simulink model "host_programa"  (R2013b)
settings: Solver=FixedStepDiscrete  StartTime=0.00000  StopTime=inf  FixedStep=0.001  MaxStep=0.001  RelTol=1e-3
undefined symbols (not defined in the file): get, hot
libraries: dsparch4 x6, dspsigops x3, dspsnks4 x1
settings Model: MAModelExclusionFile=C:\TFG\Matlab_Files\host_programa_exclusions.xml  Creator=Sr Antonio  LastModifiedBy=gonza
settings DataIOCC: LimitDataPoints=off  SaveFormat=StructureWithTime  InspectSignalLogs=on
settings OptimizationCC: ExpressionDepthLimit=2147483647
settings DebuggingCC: FcnCallInpInsideContextMsg=EnableAllAsWarning  StateNameClashWarn=warning
settings GRTTargetCC: CombineOutputUpdateFcns=off  GRTInterface=on

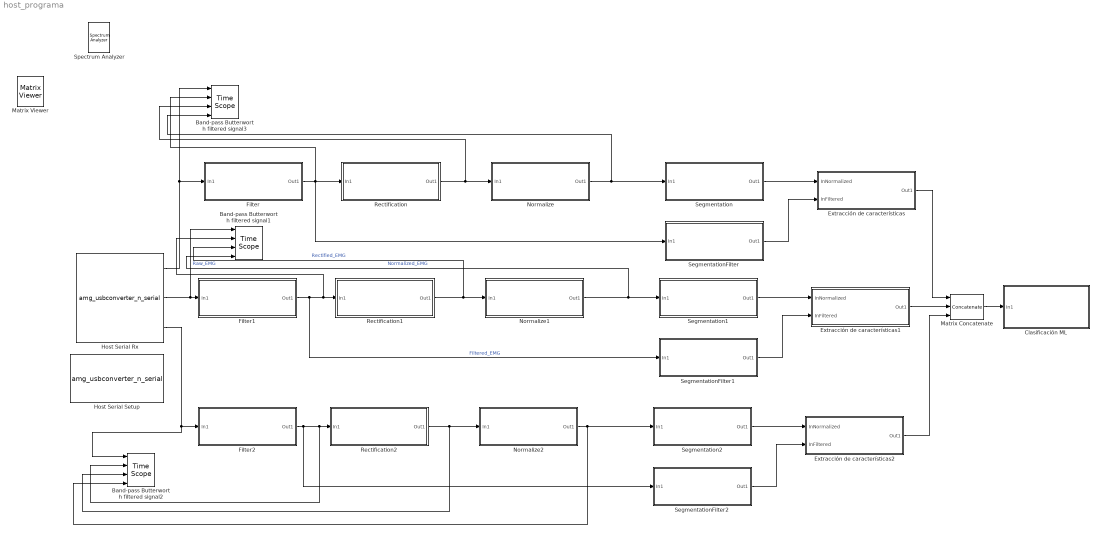
== system host_programa ==
  Band-pass Butterworth filtered signal1 : TimeScope  NumInputPorts=4  DefaultConfigurationName=spbscopes.TimeScopeBlockCfg
      settings: CopyFcn=scopeextensions.ScopeBlock.onCoreBlockCopy(gcbh);  DeleteFcn=scopeextensions.ScopeBlock.callback(gcbh, 'onBlockDelete');  PreSaveFcn=scopeextensions.ScopeBlock.callback(gcbh, 'onModelSave');  NameChangeFcn=scopeextensions.ScopeBlock.callback(gcbh, 'onBlockRename');  DestroyFcn=scopeextensions.ScopeBlock.onBlockDestroy(gcbh)  CloseFcn=scopeextensions.ScopeBlock.callback(gcbh, 'onBlockClose');  PreDeleteFcn=scopeextensions.ScopeBlock.callback(gcbh, 'onBlockPreDelete');
  Band-pass Butterworth filtered signal2 : TimeScope  NumInputPorts=4  DefaultConfigurationName=spbscopes.TimeScopeBlockCfg
      settings: CopyFcn=scopeextensions.ScopeBlock.onCoreBlockCopy(gcbh);  DeleteFcn=scopeextensions.ScopeBlock.callback(gcbh, 'onBlockDelete');  PreSaveFcn=scopeextensions.ScopeBlock.callback(gcbh, 'onModelSave');  NameChangeFcn=scopeextensions.ScopeBlock.callback(gcbh, 'onBlockRename');  DestroyFcn=scopeextensions.ScopeBlock.onBlockDestroy(gcbh)  CloseFcn=scopeextensions.ScopeBlock.callback(gcbh, 'onBlockClose');  PreDeleteFcn=scopeextensions.ScopeBlock.callback(gcbh, 'onBlockPreDelete');
  Band-pass Butterworth filtered signal3 : TimeScope  NumInputPorts=4  DefaultConfigurationName=spbscopes.TimeScopeBlockCfg
      settings: CopyFcn=scopeextensions.ScopeBlock.onCoreBlockCopy(gcbh);  DeleteFcn=scopeextensions.ScopeBlock.callback(gcbh, 'onBlockDelete');  PreSaveFcn=scopeextensions.ScopeBlock.callback(gcbh, 'onModelSave');  NameChangeFcn=scopeextensions.ScopeBlock.callback(gcbh, 'onBlockRename');  DestroyFcn=scopeextensions.ScopeBlock.onBlockDestroy(gcbh)  CloseFcn=scopeextensions.ScopeBlock.callback(gcbh, 'onBlockClose');  PreDeleteFcn=scopeextensions.ScopeBlock.callback(gcbh, 'onBlockPreDelete');
  Clasificación ML : Subsystem
  Extracción de características : Subsystem
  Extracción de características1 : Subsystem
  Extracción de características2 : Subsystem
  Filter : Subsystem
  Filter1 : Subsystem
  Filter2 : Subsystem
  Host Serial Rx : S-Function  Priority=1  FunctionName=amg_usbconverter_n_serial  Parameters=configuration,port,transfer,baudrate,stopbit,inputtype,outputtype,binheaderarray,binterminatorarray,asciiheader,asciiterminator,bindatalength,packetmode,timeout,sampletime,sampletimestr,blockid  EnableBusSupport=off  mask(amg_usbconverter_n_serial){configuration=Rx, port=COM3, baudrate=115200, databits=8, parity=None, stopbit=1, flowcontrol=None, advanceoptions=off, rxbuffersize=2048, txbuffersize=2048, transfer=Blocking, timeout=2, packetmode=Binary, binheader='0E 0E', binterminator='0A 0A', porttype_double=0, porttype_single=3, porttype_int8=0, porttype_uint8=0, porttype_int16=0, porttype_uint16=0, porttype_int32=0, porttype_uint32=0, asciiformat='%d,%f', rx_asciiterminator=LF (0x0A - "\n"), tx_asciiterminator=LF (0x0A - "\n"), inputtype=[0], outputtype=[3  1 1 1], binheaderarray=[2 14  14], binterminatorarray=[2 10  10], bindatalength=12, asciiheader=['%d,%f' uint8(10)], asciiterminator=[1 10], sampletime=0.001, sampletimestr=, blockid=HostSerialRx}
      mask prompts: baudrate "Baud rate (bps)"; databits "Data bits"; stopbit "Stop bit"; flowcontrol "Hardware flow control"; advanceoptions "Advance options"; rxbuffersize "Rx buffer size (bytes)"; txbuffersize "Tx buffer size (bytes)"; timeout "Wait time-out (Seconds)"; packetmode "Packet mode"; binheader "Binary header (example: '7E 7E')"; binterminator "Binary terminator (example: '03 03')"; porttype_double "Number of data port, type DOUBLE"; porttype_single "Number of data port, type SINGLE"; porttype_int8 "Number of data port, type INT8"; porttype_uint8 "Number of data port, type UINT8"; porttype_int16 "Number of data port, type INT16"; porttype_uint16 "Number of data port, type UINT16"; porttype_int32 "Number of data port, type INT32"; porttype_uint32 "Number of data port, type UINT32"; asciiformat "Ascii format"; rx_asciiterminator "End of packet"; tx_asciiterminator "End of packet"; inputtype "Input data type"; outputtype "Output data type"; binheaderarray "Binary header"; binterminatorarray "Binary terminator"; bindatalength "Binary data length"; asciiheader "Ascii header (printf format)"; asciiterminator "Ascii terminator"; sampletime "Sample time (sec)"; sampletimestr "Compiled sample time (sec) in string"
      mask init:
      | amg_usbconverter_n_serial_callback('init');
      mask Help: web(fullfile(waijungdocroot,'amg_usbconverter_n_uart.htm'), '-browser')
      mask TypeOptions configuration: Setup | Tx | Rx
      mask Callback configuration: amg_usbconverter_n_serial_callback('configuration');
      mask TypeOptions port: COM3
      mask Callback port: amg_usbconverter_n_serial_callback('port');
      mask Callback baudrate: amg_usbconverter_n_serial_callback('baudrate');
      mask TypeOptions databits: 8
      mask TypeOptions parity: None
      mask TypeOptions stopbit: 1 | 1.5 | 2
      mask TypeOptions flowcontrol: None | RTS | CTS | RTS/CTS
      mask Callback flowcontrol: amg_usbconverter_n_serial_callback('flowcontrol');
      mask Callback advanceoptions: amg_usbconverter_n_serial_callback('advanceoptions');
      mask TypeOptions rxbuffersize: 16 | 32 | 64 | 128 | 256 | 512 | 1024 | 2048
      mask TypeOptions txbuffersize: 16 | 32 | 64 | 128 | 256 | 512 | 1024 | 2048
      mask TypeOptions transfer: Blocking | Non-Blocking
      mask Callback transfer: amg_usbconverter_n_serial_callback('transfer');
      mask TypeOptions packetmode: Ascii | Binary
      mask Callback packetmode: amg_usbconverter_n_serial_callback('packetmode');
      mask Callback binheader: amg_usbconverter_n_serial_callback('binheader');
      mask Callback binterminator: amg_usbconverter_n_serial_callback('binterminator');
      mask Callback porttype_double: amg_usbconverter_n_serial_callback('porttype');
      mask Callback porttype_single: amg_usbconverter_n_serial_callback('porttype');
      mask Callback porttype_int8: amg_usbconverter_n_serial_callback('porttype');
      mask Callback porttype_uint8: amg_usbconverter_n_serial_callback('porttype');
      mask Callback porttype_int16: amg_usbconverter_n_serial_callback('porttype');
      mask Callback porttype_uint16: amg_usbconverter_n_serial_callback('porttype');
      mask Callback porttype_int32: amg_usbconverter_n_serial_callback('porttype');
      mask Callback porttype_uint32: amg_usbconverter_n_serial_callback('porttype');
      mask Callback asciiformat: amg_usbconverter_n_serial_callback('asciiformat');
      mask TypeOptions rx_asciiterminator: CR (0x0D - "\r") | LF (0x0A - "\n") | CRLF (0x0D 0x0A - "\r\n")
      mask Callback rx_asciiterminator: amg_usbconverter_n_serial_callback('rx_asciiterminator');
      mask TypeOptions tx_asciiterminator: CR (0x0D - "\r") | LF (0x0A - "\n") | CRLF (0x0D 0x0A - "\r\n") | None
      mask Callback tx_asciiterminator: amg_usbconverter_n_serial_callback('tx_asciiterminator');
      mask Callback sampletime: amg_usbconverter_n_serial_callback('sampletime');
      mask Callback sampletimestr: amg_usbconverter_n_serial_callback('sampletimestr');
      mask Callback blockid: amg_usbconverter_n_serial_callback('blockid');
      mask Display: text(0.05, 0.5, 'Obsolete !!!\nPort: COM3\nPacket: Binary\nTransfer: Blocking\nTs (sec): 0','ver','middle','hor','left');port_label('output', 1,'single');port_label('output', 2,'single');port_label('output', 3,'single');
  Host Serial Setup : S-Function  Priority=1  FunctionName=amg_usbconverter_n_serial  Parameters=configuration,port,transfer,baudrate,stopbit,inputtype,outputtype,binheaderarray,binterminatorarray,asciiheader,asciiterminator,bindatalength,packetmode,timeout,sampletime,sampletimestr,blockid  EnableBusSupport=off  mask(amg_usbconverter_n_serial){configuration=Setup, port=COM3, baudrate=10000000, databits=8, parity=None, stopbit=1, flowcontrol=None, advanceoptions=off, rxbuffersize=2048, txbuffersize=2048, transfer=Blocking, timeout=5, packetmode=Binary, binheader='7E 7E', binterminator='03 03', porttype_double=1, porttype_single=0, porttype_int8=1, porttype_uint8=0, porttype_int16=0, porttype_uint16=0, porttype_int32=0, porttype_uint32=0, asciiformat='%d,%f', rx_asciiterminator=CRLF (0x0D 0x0A - "\r\n"), tx_asciiterminator=CR (0x0D - "\r"), inputtype=[0], outputtype=[0], binheaderarray=[2 126  126], binterminatorarray=[2 3  3], bindatalength=0, asciiheader='', asciiterminator=[0], sampletime=inf, sampletimestr=, blockid=HostSerialSetup}
      mask prompts: baudrate "Baud rate (bps)"; databits "Data bits"; stopbit "Stop bit"; flowcontrol "Hardware flow control"; advanceoptions "Advance options"; rxbuffersize "Rx buffer size (bytes)"; txbuffersize "Tx buffer size (bytes)"; timeout "Wait time-out (Seconds)"; packetmode "Packet mode"; binheader "Binary header (example: '7E 7E')"; binterminator "Binary terminator (example: '03 03')"; porttype_double "Number of data port, type DOUBLE"; porttype_single "Number of data port, type SINGLE"; porttype_int8 "Number of data port, type INT8"; porttype_uint8 "Number of data port, type UINT8"; porttype_int16 "Number of data port, type INT16"; porttype_uint16 "Number of data port, type UINT16"; porttype_int32 "Number of data port, type INT32"; porttype_uint32 "Number of data port, type UINT32"; asciiformat "Ascii format"; rx_asciiterminator "End of packet"; tx_asciiterminator "End of packet"; inputtype "Input data type"; outputtype "Output data type"; binheaderarray "Binary header"; binterminatorarray "Binary terminator"; bindatalength "Binary data length"; asciiheader "Ascii header (printf format)"; asciiterminator "Ascii terminator"; sampletime "Sample time (sec)"; sampletimestr "Compiled sample time (sec) in string"
      mask init:
      | amg_usbconverter_n_serial_callback('init');
      mask Help: web(fullfile(waijungdocroot,'amg_usbconverter_n_uart.htm'), '-browser')
      mask TypeOptions configuration: Setup | Tx | Rx
      mask Callback configuration: amg_usbconverter_n_serial_callback('configuration');
      mask TypeOptions port: COM3
      mask Callback port: amg_usbconverter_n_serial_callback('port');
      mask Callback baudrate: amg_usbconverter_n_serial_callback('baudrate');
      mask TypeOptions databits: 8
      mask TypeOptions parity: None
      mask TypeOptions stopbit: 1 | 1.5 | 2
      mask TypeOptions flowcontrol: None | RTS | CTS | RTS/CTS
      mask Callback flowcontrol: amg_usbconverter_n_serial_callback('flowcontrol');
      mask Callback advanceoptions: amg_usbconverter_n_serial_callback('advanceoptions');
      mask TypeOptions rxbuffersize: 16 | 32 | 64 | 128 | 256 | 512 | 1024 | 2048
      mask TypeOptions txbuffersize: 16 | 32 | 64 | 128 | 256 | 512 | 1024 | 2048
      mask TypeOptions transfer: Blocking | Non-Blocking
      mask Callback transfer: amg_usbconverter_n_serial_callback('transfer');
      mask TypeOptions packetmode: Ascii | Binary
      mask Callback packetmode: amg_usbconverter_n_serial_callback('packetmode');
      mask Callback binheader: amg_usbconverter_n_serial_callback('binheader');
      mask Callback binterminator: amg_usbconverter_n_serial_callback('binterminator');
      mask Callback porttype_double: amg_usbconverter_n_serial_callback('porttype');
      mask Callback porttype_single: amg_usbconverter_n_serial_callback('porttype');
      mask Callback porttype_int8: amg_usbconverter_n_serial_callback('porttype');
      mask Callback porttype_uint8: amg_usbconverter_n_serial_callback('porttype');
      mask Callback porttype_int16: amg_usbconverter_n_serial_callback('porttype');
      mask Callback porttype_uint16: amg_usbconverter_n_serial_callback('porttype');
      mask Callback porttype_int32: amg_usbconverter_n_serial_callback('porttype');
      mask Callback porttype_uint32: amg_usbconverter_n_serial_callback('porttype');
      mask Callback asciiformat: amg_usbconverter_n_serial_callback('asciiformat');
      mask TypeOptions rx_asciiterminator: CR (0x0D - "\r") | LF (0x0A - "\n") | CRLF (0x0D 0x0A - "\r\n")
      mask Callback rx_asciiterminator: amg_usbconverter_n_serial_callback('rx_asciiterminator');
      mask TypeOptions tx_asciiterminator: CR (0x0D - "\r") | LF (0x0A - "\n") | CRLF (0x0D 0x0A - "\r\n") | None
      mask Callback tx_asciiterminator: amg_usbconverter_n_serial_callback('tx_asciiterminator');
      mask Callback sampletime: amg_usbconverter_n_serial_callback('sampletime');
      mask Callback sampletimestr: amg_usbconverter_n_serial_callback('sampletimestr');
      mask Callback blockid: amg_usbconverter_n_serial_callback('blockid');
      mask Display: text(0.5, 0.5, 'Port: COM3\nBaud (Bps): 10000000\nFrame: 8-None-1','ver','middle','hor','center');
  Matrix Concatenate : Concatenate  NumInputs=3  ConcatenateDimension=2
  Normalize : Subsystem
  Normalize1 : Subsystem
  Normalize2 : Subsystem
  Rectification : Subsystem
  Rectification1 : Subsystem
  Rectification2 : Subsystem
  Segmentation : Subsystem
  Segmentation1 : Subsystem
  Segmentation2 : Subsystem
  SegmentationFilter : Subsystem
  SegmentationFilter1 : Subsystem
  SegmentationFilter2 : Subsystem
  Matrix Viewer : dspsnks4/Matrix Viewer  IOType=viewer  ImageParams=off  CMapStr=hot(256)  AxisColorbar=on  AxisParams=off  AxisOrigin=Upper left corner  XLabel=X-axis  YLabel=Y-axis  ZLabel=Z-axis  FigPos=get(0,'defaultfigureposition')  AxisZoom=off
      settings: YMin=-1.0  YMax=1.0
  Spectrum Analyzer : SpectrumAnalyzer  IOType=viewer
      settings: CopyFcn=scopeextensions.ScopeBlock.onCoreBlockCopy(gcbh);  DeleteFcn=scopeextensions.ScopeBlock.callback(gcbh, 'onBlockDelete');  PreSaveFcn=scopeextensions.ScopeBlock.callback(gcbh, 'onModelSave');  NameChangeFcn=scopeextensions.ScopeBlock.callback(gcbh, 'onBlockRename');  DestroyFcn=scopeextensions.ScopeBlock.onBlockDestroy(gcbh)  CloseFcn=scopeextensions.ScopeBlock.callback(gcbh, 'onBlockClose');  PreDeleteFcn=scopeextensions.ScopeBlock.callback(gcbh, 'onBlockPreDelete');
  wires:
  Host Serial Rx/2 -> Band-pass Butterworth filtered signal1/1, Filter1/1(In1)  "Raw_EMG"
  Filter/1(Out1) -> SegmentationFilter/1(In1), Band-pass Butterworth filtered signal3/2, Rectification/1(In1)
  Filter1/1(Out1) -> SegmentationFilter1/1(In1), Band-pass Butterworth filtered signal1/2, Rectification1/1(In1)  "Filtered_EMG"
  Filter2/1(Out1) -> Band-pass Butterworth filtered signal2/2, Rectification2/1(In1), SegmentationFilter2/1(In1)
  Segmentation/1(Out1) -> Extracción de características/1(InNormalized)
  SegmentationFilter/1(Out1) -> Extracción de características/2(InFiltered)
  Rectification/1(Out1) -> Band-pass Butterworth filtered signal3/3, Normalize/1(In1)
  Host Serial Rx/1 -> Band-pass Butterworth filtered signal3/1, Filter/1(In1)
  Segmentation1/1(Out1) -> Extracción de características1/1(InNormalized)
  SegmentationFilter1/1(Out1) -> Extracción de características1/2(InFiltered)
  Rectification1/1(Out1) -> Band-pass Butterworth filtered signal1/3, Normalize1/1(In1)  "Rectified_EMG"
  Segmentation2/1(Out1) -> Extracción de características2/1(InNormalized)
  SegmentationFilter2/1(Out1) -> Extracción de características2/2(InFiltered)
  Rectification2/1(Out1) -> Band-pass Butterworth filtered signal2/3, Normalize2/1(In1)
  Host Serial Rx/3 -> Band-pass Butterworth filtered signal2/1, Filter2/1(In1)
  Normalize/1(Out1) -> Segmentation/1(In1), Band-pass Butterworth filtered signal3/4
  Normalize1/1(Out1) -> Band-pass Butterworth filtered signal1/4, Segmentation1/1(In1)  "Normalized_EMG"
  Normalize2/1(Out1) -> Band-pass Butterworth filtered signal2/4, Segmentation2/1(In1)
  Extracción de características/1(Out1) -> Matrix Concatenate/1
  Extracción de características1/1(Out1) -> Matrix Concatenate/2
  Extracción de características2/1(Out1) -> Matrix Concatenate/3
  Matrix Concatenate/1 -> Clasificación ML/1(In1)

== system host_programa/Clasificación ML ==
  In1 : Inport  OutDataTypeStr=double

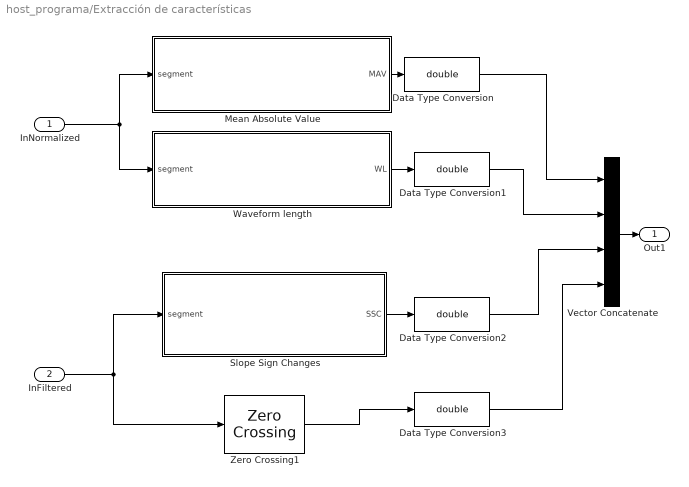
== system host_programa/Extracción de características ==
  InNormalized : Inport
  InFiltered : Inport  Port=2  OutDataTypeStr=double
  Data Type Conversion{,1..3} (4 alike) : DataTypeConversion  OutDataTypeStr=double
  Mean Absolute Value : MATLAB Function  TreatAsAtomicUnit=on
  Slope Sign Changes : MATLAB Function  TreatAsAtomicUnit=on
  Vector Concatenate : Concatenate  NumInputs=4
  Waveform length : MATLAB Function  TreatAsAtomicUnit=on
  Zero Crossing1 : dspsigops/Zero Crossing  InputProcessing=Columns as channels (frame based)
  Out1 : Outport  OutDataTypeStr=double  LockScale=on
  wires:
  InNormalized/1 -> Waveform length/1(segment), Mean Absolute Value/1(segment)
  Vector Concatenate/1 -> Out1/1
  InFiltered/1 -> Slope Sign Changes/1(segment), Zero Crossing1/1
  Mean Absolute Value/1(MAV) -> Data Type Conversion/1
  Waveform length/1(WL) -> Data Type Conversion1/1
  Slope Sign Changes/1(SSC) -> Data Type Conversion2/1
  Zero Crossing1/1 -> Data Type Conversion3/1
  Data Type Conversion/1 -> Vector Concatenate/1
  Data Type Conversion1/1 -> Vector Concatenate/2
  Data Type Conversion2/1 -> Vector Concatenate/3
  Data Type Conversion3/1 -> Vector Concatenate/4

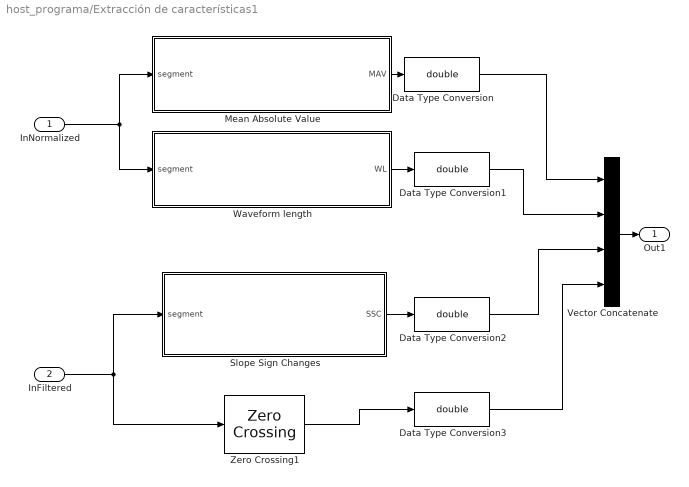
== system host_programa/Extracción de características1 ==
  InNormalized : Inport
  InFiltered : Inport  Port=2  OutDataTypeStr=double
  Data Type Conversion{,1..3} (4 alike) : DataTypeConversion  OutDataTypeStr=double
  Mean Absolute Value : MATLAB Function  TreatAsAtomicUnit=on
  Slope Sign Changes : MATLAB Function  TreatAsAtomicUnit=on
  Vector Concatenate : Concatenate  NumInputs=4
  Waveform length : MATLAB Function  TreatAsAtomicUnit=on
  Zero Crossing1 : dspsigops/Zero Crossing  InputProcessing=Columns as channels (frame based)
  Out1 : Outport  OutDataTypeStr=double  LockScale=on
  wires:
  Data Type Conversion3/1 -> Vector Concatenate/4
  Data Type Conversion2/1 -> Vector Concatenate/3
  Data Type Conversion1/1 -> Vector Concatenate/2
  Data Type Conversion/1 -> Vector Concatenate/1
  Zero Crossing1/1 -> Data Type Conversion3/1
  Slope Sign Changes/1(SSC) -> Data Type Conversion2/1
  Waveform length/1(WL) -> Data Type Conversion1/1
  Mean Absolute Value/1(MAV) -> Data Type Conversion/1
  InFiltered/1 -> Zero Crossing1/1, Slope Sign Changes/1(segment)
  Vector Concatenate/1 -> Out1/1
  InNormalized/1 -> Mean Absolute Value/1(segment), Waveform length/1(segment)

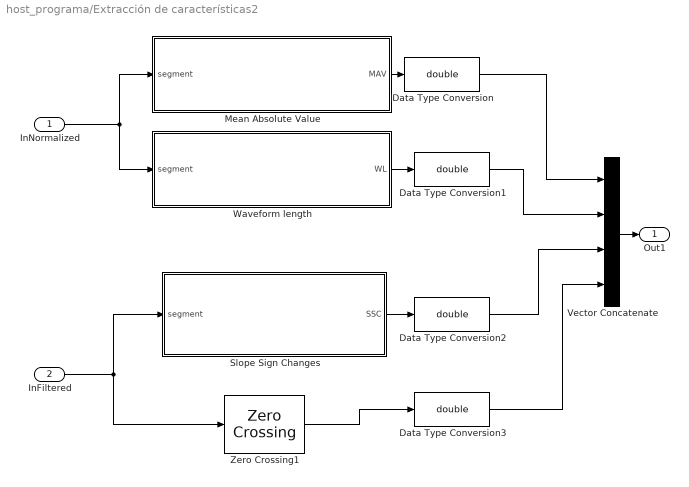
== system host_programa/Extracción de características2 ==
  InNormalized : Inport
  InFiltered : Inport  Port=2  OutDataTypeStr=double
  Data Type Conversion{,1..3} (4 alike) : DataTypeConversion  OutDataTypeStr=double
  Mean Absolute Value : MATLAB Function  TreatAsAtomicUnit=on
  Slope Sign Changes : MATLAB Function  TreatAsAtomicUnit=on
  Vector Concatenate : Concatenate  NumInputs=4
  Waveform length : MATLAB Function  TreatAsAtomicUnit=on
  Zero Crossing1 : dspsigops/Zero Crossing  InputProcessing=Columns as channels (frame based)
  Out1 : Outport  OutDataTypeStr=double  LockScale=on
  wires:
  Data Type Conversion3/1 -> Vector Concatenate/4
  Data Type Conversion2/1 -> Vector Concatenate/3
  Data Type Conversion1/1 -> Vector Concatenate/2
  Data Type Conversion/1 -> Vector Concatenate/1
  Zero Crossing1/1 -> Data Type Conversion3/1
  Slope Sign Changes/1(SSC) -> Data Type Conversion2/1
  Waveform length/1(WL) -> Data Type Conversion1/1
  Mean Absolute Value/1(MAV) -> Data Type Conversion/1
  InFiltered/1 -> Zero Crossing1/1, Slope Sign Changes/1(segment)
  Vector Concatenate/1 -> Out1/1
  InNormalized/1 -> Mean Absolute Value/1(segment), Waveform length/1(segment)

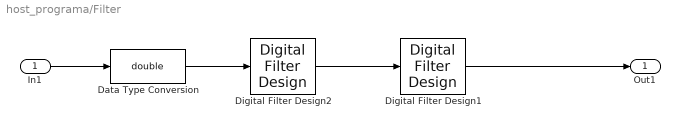
== system host_programa/Filter ==
  In1 : Inport
  Data Type Conversion : DataTypeConversion  OutDataTypeStr=double  SampleTime=0.001
  Digital Filter Design1 : dsparch4/Digital Filter Design  mwdsp_browser_bugfix_var=off
  Digital Filter Design2 : dsparch4/Digital Filter Design  mwdsp_browser_bugfix_var=off
  Out1 : Outport
  wires:
  In1/1 -> Data Type Conversion/1
  Digital Filter Design1/1 -> Out1/1
  Data Type Conversion/1 -> Digital Filter Design2/1
  Digital Filter Design2/1 -> Digital Filter Design1/1

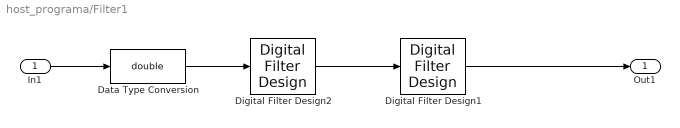
== system host_programa/Filter1 ==
  In1 : Inport
  Data Type Conversion : DataTypeConversion  OutDataTypeStr=double  SampleTime=0.001
  Digital Filter Design1 : dsparch4/Digital Filter Design  mwdsp_browser_bugfix_var=off
  Digital Filter Design2 : dsparch4/Digital Filter Design  mwdsp_browser_bugfix_var=off
  Out1 : Outport
  wires:
  Digital Filter Design2/1 -> Digital Filter Design1/1
  Data Type Conversion/1 -> Digital Filter Design2/1
  Digital Filter Design1/1 -> Out1/1
  In1/1 -> Data Type Conversion/1

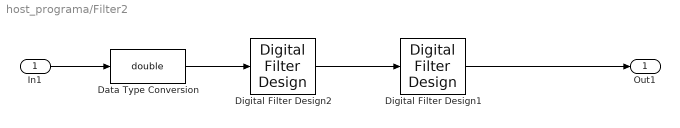
== system host_programa/Filter2 ==
  In1 : Inport
  Data Type Conversion : DataTypeConversion  OutDataTypeStr=double  SampleTime=0.001
  Digital Filter Design1 : dsparch4/Digital Filter Design  mwdsp_browser_bugfix_var=off
  Digital Filter Design2 : dsparch4/Digital Filter Design  mwdsp_browser_bugfix_var=off
  Out1 : Outport
  wires:
  Digital Filter Design2/1 -> Digital Filter Design1/1
  Data Type Conversion/1 -> Digital Filter Design2/1
  Digital Filter Design1/1 -> Out1/1
  In1/1 -> Data Type Conversion/1

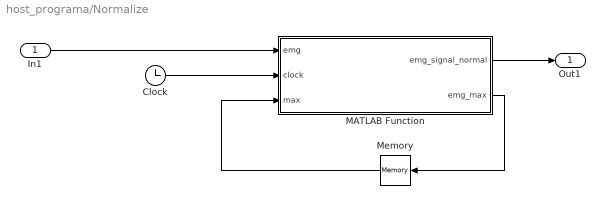
== system host_programa/Normalize ==
  In1 : Inport
  Clock : Clock
  MATLAB Function : MATLAB Function  TreatAsAtomicUnit=on
  Memory : Memory  X0=1  InheritSampleTime=on  LinearizeAsDelay=on
  Out1 : Outport
  wires:
  In1/1 -> MATLAB Function/1(emg)
  Clock/1 -> MATLAB Function/2(clock)
  MATLAB Function/2(emg_max) -> Memory/1
  Memory/1 -> MATLAB Function/3(max)
  MATLAB Function/1(emg_signal_normal) -> Out1/1

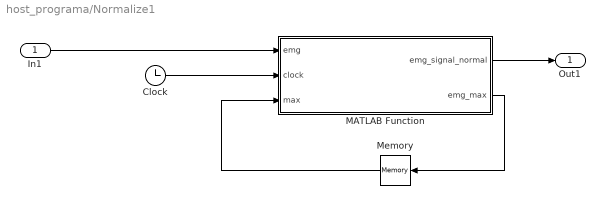
== system host_programa/Normalize1 ==
  In1 : Inport
  Clock : Clock
  MATLAB Function : MATLAB Function  TreatAsAtomicUnit=on
  Memory : Memory  X0=1  InheritSampleTime=on  LinearizeAsDelay=on
  Out1 : Outport
  wires:
  MATLAB Function/1(emg_signal_normal) -> Out1/1
  Memory/1 -> MATLAB Function/3(max)
  MATLAB Function/2(emg_max) -> Memory/1
  Clock/1 -> MATLAB Function/2(clock)
  In1/1 -> MATLAB Function/1(emg)

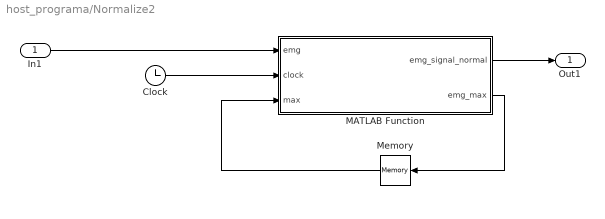
== system host_programa/Normalize2 ==
  In1 : Inport
  Clock : Clock
  MATLAB Function : MATLAB Function  TreatAsAtomicUnit=on
  Memory : Memory  X0=1  InheritSampleTime=on  LinearizeAsDelay=on
  Out1 : Outport
  wires:
  MATLAB Function/1(emg_signal_normal) -> Out1/1
  Memory/1 -> MATLAB Function/3(max)
  MATLAB Function/2(emg_max) -> Memory/1
  Clock/1 -> MATLAB Function/2(clock)
  In1/1 -> MATLAB Function/1(emg)

== system host_programa/Rectification ==
  In1 : Inport
  Abs : Abs  SampleTime=0.001  OutDataTypeStr=double
  Out1 : Outport
  wires:
  Abs/1 -> Out1/1
  In1/1 -> Abs/1  "Filtered_EMG"

== system host_programa/Rectification1 ==
  In1 : Inport
  Abs : Abs  SampleTime=0.001  OutDataTypeStr=double
  Out1 : Outport
  wires:
  In1/1 -> Abs/1  "Filtered_EMG"
  Abs/1 -> Out1/1

== system host_programa/Rectification2 ==
  In1 : Inport
  Abs : Abs  SampleTime=0.001  OutDataTypeStr=double
  Out1 : Outport
  wires:
  In1/1 -> Abs/1  "Filtered_EMG"
  Abs/1 -> Out1/1

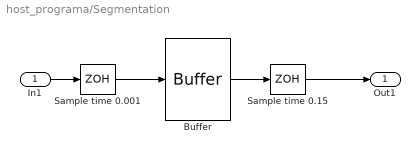
== system host_programa/Segmentation ==
  In1 : Inport
  Buffer : Buffer  N=200  V=50  TreatMby1Signals=One channel
  Sample time 0.001 : ZeroOrderHold  SampleTime=0.001
  Sample time 0.15 : ZeroOrderHold  SampleTime=0.15
  Out1 : Outport
  wires:
  Sample time 0.001/1 -> Buffer/1
  In1/1 -> Sample time 0.001/1
  Sample time 0.15/1 -> Out1/1
  Buffer/1 -> Sample time 0.15/1

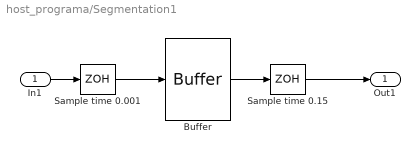
== system host_programa/Segmentation1 ==
  In1 : Inport
  Buffer : Buffer  N=200  V=50  TreatMby1Signals=One channel
  Sample time 0.001 : ZeroOrderHold  SampleTime=0.001
  Sample time 0.15 : ZeroOrderHold  SampleTime=0.15
  Out1 : Outport
  wires:
  Buffer/1 -> Sample time 0.15/1
  Sample time 0.15/1 -> Out1/1
  In1/1 -> Sample time 0.001/1
  Sample time 0.001/1 -> Buffer/1

== system host_programa/Segmentation2 ==
  In1 : Inport
  Buffer : Buffer  N=200  V=50  TreatMby1Signals=One channel
  Sample time 0.001 : ZeroOrderHold  SampleTime=0.001
  Sample time 0.15 : ZeroOrderHold  SampleTime=0.15
  Out1 : Outport
  wires:
  Buffer/1 -> Sample time 0.15/1
  Sample time 0.15/1 -> Out1/1
  In1/1 -> Sample time 0.001/1
  Sample time 0.001/1 -> Buffer/1

== system host_programa/SegmentationFilter ==
  In1 : Inport
  Buffer : Buffer  N=200  V=50  TreatMby1Signals=One channel
  Sample time 0.001 : ZeroOrderHold  SampleTime=0.001
  Sample time 0.15 : ZeroOrderHold  SampleTime=0.15
  Out1 : Outport
  wires:
  Buffer/1 -> Sample time 0.15/1
  Sample time 0.15/1 -> Out1/1
  In1/1 -> Sample time 0.001/1
  Sample time 0.001/1 -> Buffer/1

== system host_programa/SegmentationFilter1 ==
  In1 : Inport
  Buffer : Buffer  N=200  V=50  TreatMby1Signals=One channel
  Sample time 0.001 : ZeroOrderHold  SampleTime=0.001
  Sample time 0.15 : ZeroOrderHold  SampleTime=0.15
  Out1 : Outport
  wires:
  Sample time 0.001/1 -> Buffer/1
  In1/1 -> Sample time 0.001/1
  Sample time 0.15/1 -> Out1/1
  Buffer/1 -> Sample time 0.15/1

== system host_programa/SegmentationFilter2 ==
  In1 : Inport
  Buffer : Buffer  N=200  V=50  TreatMby1Signals=One channel
  Sample time 0.001 : ZeroOrderHold  SampleTime=0.001
  Sample time 0.15 : ZeroOrderHold  SampleTime=0.15
  Out1 : Outport
  wires:
  Sample time 0.001/1 -> Buffer/1
  In1/1 -> Sample time 0.001/1
  Sample time 0.15/1 -> Out1/1
  Buffer/1 -> Sample time 0.15/1

== matlab function host_programa/Normalize/MATLAB Function ==
  data: emg input; emg_signal_normal output; clock input; max input; emg_max output
function [emg_signal_normal, emg_max] = fcn(emg, clock, max)
%% Output
%emg_signal_normal: Valor de la señal de EMG normalizado
%emg_max: Valor máximo de amplitud de la EMG en t-1
%% Input
%emg: Señal de EMG de entrada (Rectificada)
%clock: Tiempo de simulación
%max: Valor máximo de amplitud de la EMG en t
%% Ignorar los primeros 2 segundos de señal
if clock <= 2
    emg_signal_normal = 0;
    emg_max = 0;
    
else
    %% Coger el valor máximo de amplitud durante los 18 segundos restantes
    if clock <= 20
        emg_signal_normal = 0;
        if emg > max
            emg_max = emg;
        else
            emg_max = max;
        end
        %% Normalizar el valor de la señal de entrada
    else
        emg_signal_normal = emg/max;
        %% Tomar el valor máximo en t como el proximo valor máximo en t-1 y realimentar con el la función
        emg_max = max;
    end
end

== matlab function host_programa/Extracción de características/Mean Absolute Value ==
  data: segment input; MAV output
function MAV = MeanAbsoluteValue(segment)
    L = length(segment);
    S = sum(abs(segment));
    MAV = S/L;
end

== matlab function host_programa/Extracción de características/Waveform length ==
  data: segment input; WL output
function WL = WaveformLength(segment)
    WL = 0;
    L = length(segment);
    for i = 1:(L-1)
        WL = WL + (segment(i+1)-segment(i));
    end
end

== matlab function host_programa/Extracción de características1/Mean Absolute Value ==
  data: segment input; MAV output
function MAV = MeanAbsoluteValue(segment)
    L = length(segment);
    S = sum(abs(segment));
    MAV = S/L;
end

== matlab function host_programa/Extracción de características/Slope Sign Changes ==
  data: segment input; SSC output
function SSC = SlopeSignChanges(segment)
SSC = 0;
L = length(segment);
for i = 2:(L-1)
    if (segment(i) > segment(i-1)) && (segment(i) > segment(i+1))
        SSC = SSC + 1;
    end
    if (segment(i) < segment(i-1)) && (segment(i) < segment(i+1))
        SSC = SSC + 1;
    end
end
end

== matlab function host_programa/Extracción de características1/Slope Sign Changes ==
  data: segment input; SSC output
function SSC = SlopeSignChanges(segment)
SSC = 0;
L = length(segment);
for i = 2:(L-1)
    if (segment(i) > segment(i-1)) && (segment(i) > segment(i+1))
        SSC = SSC + 1;
    end
    if (segment(i) < segment(i-1)) && (segment(i) < segment(i+1))
        SSC = SSC + 1;
    end
end
end

== matlab function host_programa/Extracción de características1/Waveform length ==
  data: segment input; WL output
function WL = WaveformLength(segment)
    WL = 0;
    L = length(segment);
    for i = 1:(L-1)
        WL = WL + (segment(i+1)-segment(i));
    end
end

== matlab function host_programa/Normalize1/MATLAB Function ==
  data: emg input; emg_signal_normal output; clock input; max input; emg_max output
function [emg_signal_normal, emg_max] = fcn(emg, clock, max)
%% Output
%emg_signal_normal: Valor de la señal de EMG normalizado
%emg_max: Valor máximo de amplitud de la EMG en t-1
%% Input
%emg: Señal de EMG de entrada (Rectificada)
%clock: Tiempo de simulación
%max: Valor máximo de amplitud de la EMG en t
%% Ignorar los primeros 2 segundos de señal
if clock <= 2
    emg_signal_normal = 0;
    emg_max = 0;
    
else
    %% Coger el valor máximo de amplitud durante los 18 segundos restantes
    if clock <= 20
        emg_signal_normal = 0;
        if emg > max
            emg_max = emg;
        else
            emg_max = max;
        end
        %% Normalizar el valor de la señal de entrada
    else
        emg_signal_normal = emg/max;
        %% Tomar el valor máximo en t como el proximo valor máximo en t-1 y realimentar con el la función
        emg_max = max;
    end
end

== matlab function host_programa/Extracción de características2/Mean Absolute Value ==
  data: segment input; MAV output
function MAV = MeanAbsoluteValue(segment)
    L = length(segment);
    S = sum(abs(segment));
    MAV = S/L;
end

== matlab function host_programa/Extracción de características2/Slope Sign Changes ==
  data: segment input; SSC output
function SSC = SlopeSignChanges(segment)
SSC = 0;
L = length(segment);
for i = 2:(L-1)
    if (segment(i) > segment(i-1)) && (segment(i) > segment(i+1))
        SSC = SSC + 1;
    end
    if (segment(i) < segment(i-1)) && (segment(i) < segment(i+1))
        SSC = SSC + 1;
    end
end
end

== matlab function host_programa/Extracción de características2/Waveform length ==
  data: segment input; WL output
function WL = WaveformLength(segment)
    WL = 0;
    L = length(segment);
    for i = 1:(L-1)
        WL = WL + (segment(i+1)-segment(i));
    end
end

== matlab function host_programa/Normalize2/MATLAB Function ==
  data: emg input; emg_signal_normal output; clock input; max input; emg_max output
function [emg_signal_normal, emg_max] = fcn(emg, clock, max)
%% Output
%emg_signal_normal: Valor de la señal de EMG normalizado
%emg_max: Valor máximo de amplitud de la EMG en t-1
%% Input
%emg: Señal de EMG de entrada (Rectificada)
%clock: Tiempo de simulación
%max: Valor máximo de amplitud de la EMG en t
%% Ignorar los primeros 2 segundos de señal
if clock <= 2
    emg_signal_normal = 0;
    emg_max = 0;
    
else
    %% Coger el valor máximo de amplitud durante los 18 segundos restantes
    if clock <= 20
        emg_signal_normal = 0;
        if emg > max
            emg_max = emg;
        else
            emg_max = max;
        end
        %% Normalizar el valor de la señal de entrada
    else
        emg_signal_normal = emg/max;
        %% Tomar el valor máximo en t como el proximo valor máximo en t-1 y realimentar con el la función
        emg_max = max;
    end
end
